simulink model "Val_Rec"  (Simulink 7.1)
settings: Solver=ode4  StartTime=0.0  StopTime=6  FixedStep=0.01  RelTol=1e-3
undefined symbols (not defined in the file or in its folder): cinvMitsu, Dterminante, pol5Grx, pol5Gry, pol5Grz, secuenciax, secuenciay, secuenciaz
libraries: simulink x3
settings Model: Creator=Dario  LastModifiedBy=Dario

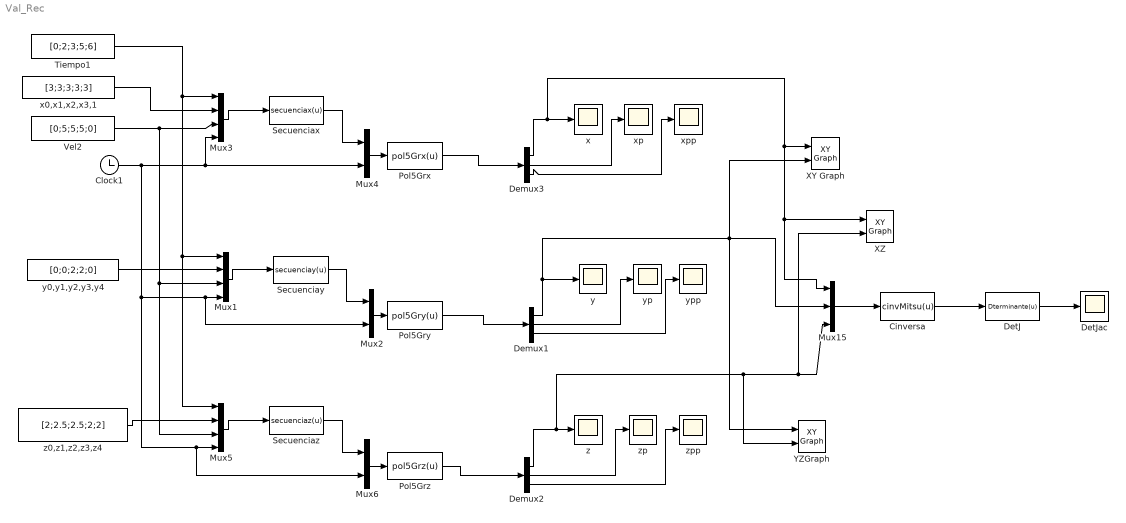
== system Val_Rec ==
  Cinversa : MATLABFcn  MATLABFcn=cinvMitsu(u)  OutputDimensions=3
  Clock1 : Clock
      settings: Decimation=10
  Demux1 : Demux  Outputs=3
  Demux2 : Demux  Outputs=3
  Demux3 : Demux  Outputs=3
  DetJ : MATLABFcn  MATLABFcn=Dterminante(u)  OutputDimensions=1
  DetJac : Scope
      settings: YMin=-9.21924  YMax=-9.21924  SaveName=ScopeData9
  Mux1 : Mux
  Mux15 : Mux  Inputs=3
  Mux2 : Mux  Inputs=2
  Mux3 : Mux
  Mux4 : Mux  Inputs=2
  Mux5 : Mux
  Mux6 : Mux  Inputs=2
  Pol5Grx : MATLABFcn  MATLABFcn=pol5Grx(u)  OutputDimensions=3
  Pol5Gry : MATLABFcn  MATLABFcn=pol5Gry(u)  OutputDimensions=3
  Pol5Grz : MATLABFcn  MATLABFcn=pol5Grz(u)  OutputDimensions=3
  Secuenciax : MATLABFcn  MATLABFcn=secuenciax(u)  OutputDimensions=6
  Secuenciay : MATLABFcn  MATLABFcn=secuenciay(u)  OutputDimensions=6
  Secuenciaz : MATLABFcn  MATLABFcn=secuenciaz(u)  OutputDimensions=6
  Tiempo1 : Constant  Value=[0;2;3;5;6]  OutDataType=sfix(16)  OutScaling=2^0
  Vel2 : Constant  Value=[0;5;5;5;0]  OutDataType=sfix(16)  OutScaling=2^0
  XY Graph : simulink/Sinks/XY Graph  SystemSampleTime=-1  xmin=-10  xmax=10  ymin=-10  ymax=10  st=-1
  XZ : simulink/Sinks/XY Graph  SystemSampleTime=-1  xmin=-10  xmax=10  ymin=-10  ymax=10  st=-1
  YZGraph : simulink/Sinks/XY Graph  SystemSampleTime=-1  xmin=-10  xmax=10  ymin=-10  ymax=10  st=-1
  x : Scope
      settings: SaveName=ScopeData6
  x0,x1,x2,x3,1 : Constant  Value=[3;3;3;3;3]  OutDataType=sfix(16)  OutScaling=2^0
  xp : Scope
      settings: SaveName=ScopeData7
  xpp : Scope
      settings: SaveName=ScopeData8
  y : Scope
  y0,y1,y2,y3,y4 : Constant  Value=[0;0;2;2;0]  OutDataType=sfix(16)  OutScaling=2^0
  yp : Scope
  ypp : Scope
      settings: SaveName=ScopeData2
  z : Scope
      settings: SaveName=ScopeData3
  z0,z1,z2,z3,z4 : Constant  Value=[2;2.5;2.5;2;2]  OutDataType=sfix(16)  OutScaling=2^0
  zp : Scope
      settings: SaveName=ScopeData4
  zpp : Scope
      settings: SaveName=ScopeData5
  wires:
  Mux3/1 -> Secuenciax/1
  Tiempo1/1 -> Mux3/1, Mux1/1, Mux5/1
  x0,x1,x2,x3,1/1 -> Mux3/2
  Clock1/1 -> Mux3/4, Mux4/2, Mux1/4, Mux2/2, Mux5/4, Mux6/2
  Mux4/1 -> Pol5Grx/1
  Vel2/1 -> Mux3/3, Mux1/3, Mux5/3
  Secuenciax/1 -> Mux4/1
  Pol5Grx/1 -> Demux3/1
  Demux3/1 -> x/1, XY Graph/1, XZ/1, Mux15/1
  Demux3/2 -> xp/1
  Demux3/3 -> xpp/1
  Mux1/1 -> Secuenciay/1
  y0,y1,y2,y3,y4/1 -> Mux1/2
  Mux2/1 -> Pol5Gry/1
  Secuenciay/1 -> Mux2/1
  Pol5Gry/1 -> Demux1/1
  Demux1/1 -> y/1, XY Graph/2, YZGraph/1, Mux15/2
  Demux1/2 -> yp/1
  Demux1/3 -> ypp/1
  Mux5/1 -> Secuenciaz/1
  z0,z1,z2,z3,z4/1 -> Mux5/2
  Mux6/1 -> Pol5Grz/1
  Secuenciaz/1 -> Mux6/1
  Pol5Grz/1 -> Demux2/1
  Demux2/1 -> z/1, YZGraph/2, XZ/2, Mux15/3
  Demux2/2 -> zp/1
  Demux2/3 -> zpp/1
  Mux15/1 -> Cinversa/1
  Cinversa/1 -> DetJ/1
  DetJ/1 -> DetJac/1
